simulink model "earth_model"  (R2014b)
settings: Solver=ode3  StartTime=0.0  StopTime=10.0  FixedStep=dt  RelTol=1e-3
values from neighbouring files (symbols this model uses):
  dt = 1    [earth_model_run.m]
settings Model: Creator=root  LastModifiedBy=root
settings DataIOCC: SaveOutput=off  SaveTime=off

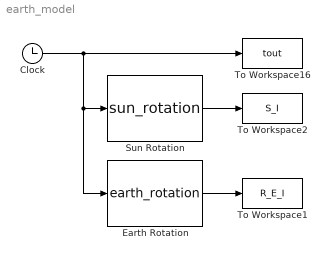
== system earth_model ==
  Clock : Clock
  Earth Rotation : MATLABFcn  MATLABFcn=earth_rotation  OutputDimensions=[3,3]  Output1D=off
  Sun Rotation : MATLABFcn  MATLABFcn=sun_rotation  OutputDimensions=[3,1]  Output1D=off
  To Workspace1 : ToWorkspace  VariableName=R_E_I  SampleTime=dt
  To Workspace16 : ToWorkspace  VariableName=tout  SampleTime=dt
  To Workspace2 : ToWorkspace  VariableName=S_I  SampleTime=dt
  wires:
  Sun Rotation/1 -> To Workspace2/1
  Clock/1 -> Sun Rotation/1, Earth Rotation/1, To Workspace16/1
  Earth Rotation/1 -> To Workspace1/1
